simulink library "Thermosyphon"  (R2018b)
settings: Solver=ode45  StartTime=0.0  StopTime=10.0  RelTol=1e-3  EnableMultiTasking=on
undefined symbols (not defined in the file): MassFlow, Temperature, Water
libraries: carnot x2, simulink x1
settings Model: Creator=Hafner  LastModifiedBy=drhf
settings DataIOCC: LimitDataPoints=on  SaveFormat=Array  SignalLoggingSaveFormat=ModelDataLogs
settings OptimizationCC: ExpressionDepthLimit=2147483647  LifeSpan=inf
settings DebuggingCC: UnderspecifiedInitializationDetection=Classic  MergeDetectMultiDrivingBlocksExec=none  SolverPrmCheckMsg=warning  FcnCallInpInsideContextMsg=warning  StateNameClashWarn=warning  SFUnexpectedBacktrackingDiag=warning  SFNoUnconditionalDefaultTransitionDiag=warning  SFExecutionAtInitializationDiag=none
settings HardwareCC: ProdBitPerPointer=32  ProdBitPerSizeT=32  ProdBitPerPtrDiffT=32  ProdLargestAtomicFloat=None  ProdIntDivRoundTo=Undefined  ProdEndianess=Unspecified  ProdWordSize=32  ProdHWDeviceType=32-bit Generic
settings ModelReferenceCC: PropagateSignalLabelsOutOfModel=off
settings SFSimCC: SimUseLocalCustomCode=off
settings RTWCC: RTWUseLocalCustomCode=off
settings CodeAppCC: StateflowObjectComments=on
settings GRTTargetCC: TargetLangStandard=C89/C90 (ANSI)  GeneratePreprocessorConditionals=Disable all  CombineOutputUpdateFcns=off  GRTInterface=on
settings ConfigComp: CovMetricSettings=dw  CovHtmlReporting=on  CovSaveCumulativeToWorkspaceVar=on  CovSaveSingleToWorkspaceVar=on  CovExternalEMLEnable=off

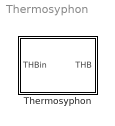
== system Thermosyphon ==
  Thermosyphon : Subsystem  mask(thermosyphon){p0=3e5, dia=0.025, fluid_id=Water, mix=0, mix2=0, mix3=0, t1=1}
      mask prompts: p0 "static system pressure [Pa]"; dia "Diameter at in- and outlet [m]"; fluid_id "fluid"; mix "fluid mixture [0..1]"; mix2 "fluid mixture 2 [0..1]"; mix3 "fluid mixture 3 [0..1]"; t1 "Time constant of PT1 transfer function for massflow in s"
      mask help:
      | This block is a model of a "thermosyphon pump". Place it in natural convection systems as you would place a pump.
      | Assure that the sum of heights is zero. Otherwise the simulation will not start.
      | You may check the sum of heights by verifying the "Geodetic Height" in the THB at the inport of this block.
      | If the sum is not zero, the difference is displayed in the subsystem "Stop Simulation".
      | This model uses a Memory block to break an algebraic loop. Avoid using the variable-step solver ode15s or ode113 (see block help for details).
      | A unit delay block with a sample time ("time constant of the pump") limits the maximum stepsize.
      mask Help: web(fullfile(path_carnot('help'),'Thermosyphon.html'),'-helpbrowser')
      mask TypeOptions p0: basic_THB/p
      mask TypeOptions dia: basic_THB/dia
      mask TypeOptions fluid_id: basic_THB/fluid
      mask TypeOptions mix: basic_THB/mix
      mask TypeOptions mix2: basic_THB/mix2
      mask TypeOptions mix3: basic_THB/mix3
      mask TypeOptions t1: Transfer Fcn/t1
      mask DialogControl Container4 Prompt: Hydraulic
      mask Display: plot(0,0,100,100,[90,10],[80,90],[90,10],[70,80],[90,10],[20,10],[90,10],[30,20],[40,60,40,40],[60,50,40,60])

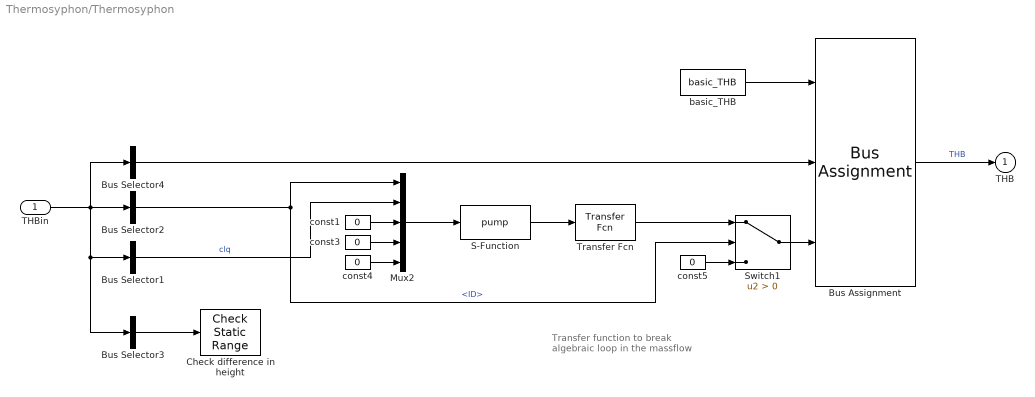
== system Thermosyphon/Thermosyphon ==
  note: Transfer function to
      | break algebraic loop
      | in the massflow
  THBin : Inport
  Bus Assignment : BusAssignment  AssignedSignals=Temperature,MassFlow
  Bus Selector1 : BusSelector  OutputSignals=DPConstant,DPLinear,DPQuadratic  OutputAsBus=on
  Bus Selector2 : BusSelector  OutputSignals=ID
  Bus Selector3 : BusSelector  OutputSignals=GeodeticHeight  OutputAsBus=on
  Bus Selector4 : BusSelector  OutputSignals=Temperature  OutputAsBus=on
  Check difference in height : simulink/Model Verification/Check  Static Range  Description=-0.001 <= u <= 0.001  max=0.001  max_included=on  min=-0.001  min_included=on  enabled=on  stopWhenAssertionFail=on  export=off  icon=graphic
      settings: SourceProductName=Simulink  SourceProductBaseCode=SL
  Mux2 : Mux  Inputs=5
  S-Function : S-Function  FunctionName=pump  SFunctionDeploymentMode=off  EnableBusSupport=off
  Switch1 : Switch  Criteria=u2 > Threshold  SaturateOnIntegerOverflow=on  InputSameDT=on
  Transfer Fcn : carnot/Hydraulics/Pump_Main/Transfer Fcn  t1=t1
      settings: SourceProductName=Carnot
  basic_THB : carnot/Basic/Hydraulics/basic_THB  t=20  mdot=0  p=p0  ID=Full Pressure Drop with Static Height  fluid=Water  mix=mix  mix2=mix2  mix3=mix3  dia=dia  hgt=0
      settings: SourceProductName=Carnot
  const{1,3..5} (4 alike) : Constant  Value=0
  THB : Outport
  wires:
  Bus Selector4/1 -> Bus Assignment/2
  Bus Selector2/1 -> Mux2/1, Switch1/2  "<ID>"
  Mux2/1 -> S-Function/1
  S-Function/1 -> Transfer Fcn/1
  const3/1 -> Mux2/4
  const4/1 -> Mux2/5
  const1/1 -> Mux2/3
  Transfer Fcn/1 -> Switch1/1
  const5/1 -> Switch1/3
  basic_THB/1 -> Bus Assignment/1
  Bus Assignment/1 -> THB/1  "THB"
  Bus Selector1/1 -> Mux2/2  "clq"
  THBin/1 -> Bus Selector2/1, Bus Selector1/1, Bus Selector3/1, Bus Selector4/1
  Switch1/1 -> Bus Assignment/3
  Bus Selector3/1 -> Check difference in height/1
